simulink model "spike_generator"  (R2020b)
settings: Solver=FixedStepDiscrete  StartTime=0.0  StopTime=stopTime  RelTol=1e-3
InitFcn:
  | initCallback
StopFcn:
  | stopCallback
values from neighbouring files (symbols this model uses):
  nSites = 4    [modelparameters.m]
  t_rd_init = t_rd_rest + 0.02e-3*spont - t_rd_jump    (= 0.0156)    [modelparameters.m]
  t_rd_jump = 0.4e-3    (= 0.0004)    [modelparameters.m]
  t_rd_rest = 14.0e-3    (= 0.014)    [modelparameters.m]
  tabs = 10e-3    (= 0.01)    [modelparameters.m]
  tau = 60e-3    (= 0.06)    [modelparameters.m]
  tdres = 1/Fs    (= 2.08333333333e-05)    [modelparameters.m]
  trel = 10e-3    (= 0.01)    [modelparameters.m]
undefined symbols (not defined in the file or in its folder): mp
libraries: hdlsllib x13
settings Model: Creator=Ross  LastModifiedBy=tyler
settings SolverCC: AutoInsertRateTranBlk=on
settings DataIOCC: SaveOutput=off  SaveTime=off  ReturnWorkspaceOutputs=off
settings OptimizationCC: BlockReduction=off  ConditionallyExecuteInputs=off  DefaultParameterBehavior=Inlined
settings DebuggingCC: ReadBeforeWriteMsg=DisableAll  WriteAfterWriteMsg=DisableAll  WriteAfterReadMsg=DisableAll  AlgebraicLoopMsg=error  MultiTaskDSMMsg=none  SingleTaskRateTransMsg=error  PregeneratedLibrarySubsystemCodeDiagnostic=none  ArithmeticOperatorsInVariantConditions=warning
settings HardwareCC: ProdBitPerPointer=32  ProdBitPerSizeT=32  ProdBitPerPtrDiffT=32  ProdLargestAtomicFloat=None  ProdIntDivRoundTo=Undefined  ProdEndianess=Unspecified  ProdWordSize=32  ProdHWDeviceType=ASIC/FPGA->ASIC/FPGA  TargetBitPerPointer=64  TargetBitPerSizeT=64  TargetBitPerPtrDiffT=64  TargetLongLongMode=on  TargetIntDivRoundTo=Zero  TargetEndianess=LittleEndian  TargetWordSize=64  TargetHWDeviceType=Custom Processor->MATLAB Host Computer  ProdEqTarget=off
settings ModelReferenceCC: UpdateModelReferenceTargets=IfOutOfDate  ModelReferenceNumInstancesAllowed=Single
settings SFSimCC: SFSimEcho=off  SimUseLocalCustomCode=off  CustomCodeUndefinedFunction=UseInterfaceOnly
settings RTWCC: RTWUseLocalCustomCode=off

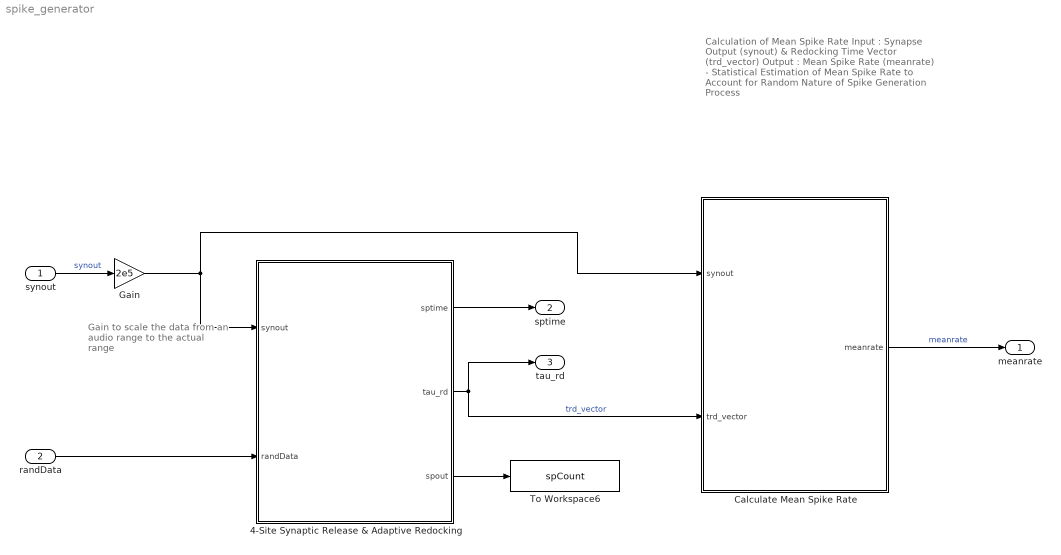
== system spike_generator ==
  note: Gain to scale the
      | data from an audio
      | range to the actual
      | range
  note: Calculation of Mean Spike Rate
      |
      | Input : Synapse Output (synout) & Redocking Time Vector (trd_vector)
      |
      | Output : Mean Spike Rate (meanrate)
      |
      | - Statistical Estimation of Mean Spike Rate to Account for Random Nature of Spike Generation Process
  synout : Inport  OutDataTypeStr=single  PortDimensions=1  SampleTime=[2.0833333333333333e-05,0]
  randData : Inport  Port=2  OutDataTypeStr=single  PortDimensions=[1 1]  SampleTime=[2.0833333333333333e-05,0]
  4-Site Synaptic Release & Adaptive Redocking : Subsystem
  Calculate Mean Spike Rate : Subsystem
  Gain : Gain  Gain=2e5
  To Workspace6 : ToWorkspace  VariableName=spCount  SampleTime=-1
      settings: Save2DSignal=2-D array (concatenate along first dimension)
  meanrate : Outport  OutDataTypeStr=single  PortDimensions=1  SampleTime=[2.0833333333333333e-05,0]
  sptime : Outport  Port=2  OutDataTypeStr=single  PortDimensions=1  SampleTime=[2.0833333333333333e-05,0]
  tau_rd : Outport  Port=3  OutDataTypeStr=single  PortDimensions=1  SampleTime=[2.0833333333333333e-05,0]
  wires:
  4-Site Synaptic Release & Adaptive Redocking/2(tau_rd) -> Calculate Mean Spike Rate/2(trd_vector), tau_rd/1  "trd_vector"
  Calculate Mean Spike Rate/1(meanrate) -> meanrate/1  "meanrate"
  randData/1 -> 4-Site Synaptic Release & Adaptive Redocking/2(randData)
  4-Site Synaptic Release & Adaptive Redocking/1(sptime) -> sptime/1
  synout/1 -> Gain/1  "synout"
  Gain/1 -> 4-Site Synaptic Release & Adaptive Redocking/1(synout), Calculate Mean Spike Rate/1(synout)
  4-Site Synaptic Release & Adaptive Redocking/3(spout) -> To Workspace6/1

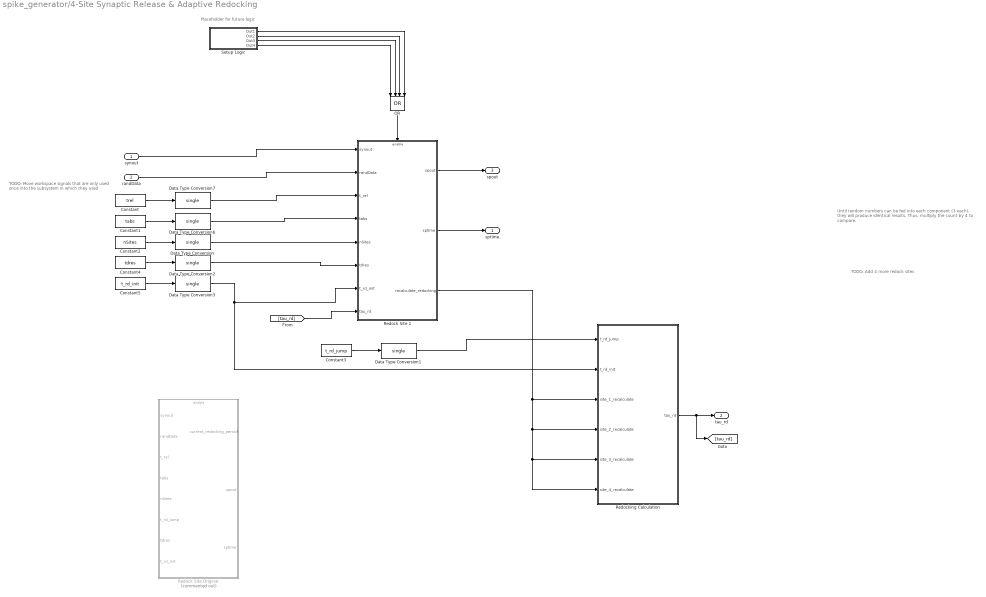
== system spike_generator/4-Site Synaptic Release & Adaptive Redocking ==
  note: TODO: Add 4 more redock sites
  note: Until random numbers can be fed into each component (3 each),
      |  they will produce identical results.  Thus, multiply the count by
      | 4 to compare.
  note: TODO: Move workspace signals that are only
      | used once into the subsystem in which they
      | used
  note: Placeholder for future logic
  synout : Inport
  randData : Inport  Port=2
  Constant : Constant  Value=trel  SampleTime=mp.Ts_sim
  Constant1 : Constant  Value=tabs  SampleTime=mp.Ts_sim
  Constant2 : Constant  Value=nSites  SampleTime=mp.Ts_sim
  Constant3 : Constant  Value=t_rd_jump  SampleTime=mp.Ts_sim
  Constant4 : Constant  Value=tdres  SampleTime=mp.Ts_sim
  Constant5 : Constant  Value=t_rd_init  SampleTime=mp.Ts_sim
  Data Type Conversion{,1..3,6..7} (6 alike) : DataTypeConversion  OutDataTypeStr=single  RndMeth=Nearest
  OR : Logic  Operator=OR  Inputs=4  IconShape=distinctive  AllPortsSameDT=off  OutDataTypeStr=boolean
  Redock Site 1 : Subsystem  TreatAsAtomicUnit=on
  Redock Site Original : Subsystem  Commented=on  TreatAsAtomicUnit=on
  Redocking Calculation : Subsystem
  Setup Logic : Subsystem
  sptime : Outport
  tau_rd : Outport  Port=2
  spout : Outport  Port=3
  wires:
  Setup Logic/1(Out1) -> OR/4
  Setup Logic/2(Out2) -> OR/3
  Setup Logic/3(Out3) -> OR/2
  Setup Logic/4(Out4) -> OR/1
  OR/1 -> Redock Site 1/Enable
  Constant5/1 -> Data Type Conversion3/1
  Constant4/1 -> Data Type Conversion2/1
  Constant3/1 -> Data Type Conversion1/1
  Constant2/1 -> Data Type Conversion/1
  Constant1/1 -> Data Type Conversion6/1
  Data Type Conversion6/1 -> Redock Site 1/4(tabs)
  Data Type Conversion7/1 -> Redock Site 1/3(t_rel)
  Constant/1 -> Data Type Conversion7/1
  Data Type Conversion3/1 -> Redocking Calculation/2(t_rd_init), Redock Site 1/7(t_rd_init)
  Data Type Conversion2/1 -> Redock Site 1/6(tdres)
  Data Type Conversion1/1 -> Redocking Calculation/1(t_rd_jump)
  Data Type Conversion/1 -> Redock Site 1/5(nSites)
  randData/1 -> Redock Site 1/2(randData)
  synout/1 -> Redock Site 1/1(synout)
  Redock Site 1/2(sptime) -> sptime/1
  Redock Site 1/1(spout) -> spout/1
  Redocking Calculation/1(tau_rd) -> tau_rd/1, [tau_rd]
  [tau_rd] -> Redock Site 1/8(tau_rd)
  Redock Site 1/3(recalculate_redocking) -> Redocking Calculation/5(site_3_recalculate), Redocking Calculation/6(site_4_recalculate), Redocking Calculation/4(site_2_recalculate), Redocking Calculation/3(site_1_recalculate)

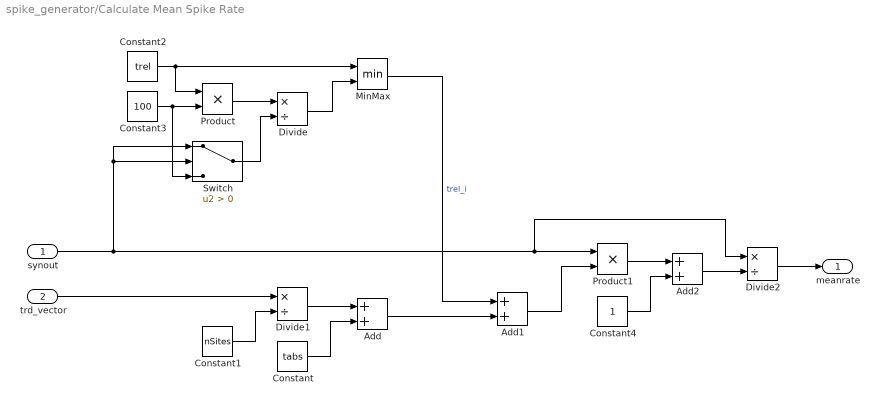
== system spike_generator/Calculate Mean Spike Rate ==
  synout : Inport
  trd_vector : Inport  Port=2
  Add : Sum
  Add1 : Sum
  Add2 : Sum
  Constant : Constant  Value=tabs  OutDataTypeStr=single  SampleTime=-1
  Constant1 : Constant  Value=nSites  OutDataTypeStr=single  SampleTime=-1
  Constant2 : Constant  Value=trel  OutDataTypeStr=single  SampleTime=-1
  Constant3 : Constant  Value=100  OutDataTypeStr=single  SampleTime=-1
  Constant4 : Constant  OutDataTypeStr=single  SampleTime=-1
  Divide : Product  Inputs=*/  RndMeth=Zero  SaturateOnIntegerOverflow=on
  Divide1 : Product  Inputs=*/  RndMeth=Zero  SaturateOnIntegerOverflow=on
  Divide2 : Product  Inputs=*/  RndMeth=Zero  SaturateOnIntegerOverflow=on
  MinMax : MinMax  Inputs=2
  Product : Product
  Product1 : Product
  Switch : Switch  Criteria=u2 > Threshold
  meanrate : Outport  VectorParamsAs1DForOutWhenUnconnected=off
  wires:
  Switch/1 -> Divide/2
  Divide2/1 -> meanrate/1
  Add2/1 -> Divide2/2
  Product1/1 -> Add2/1
  Add1/1 -> Product1/2
  Constant4/1 -> Add2/2
  Add/1 -> Add1/2
  Constant/1 -> Add/2
  Divide1/1 -> Add/1
  Constant1/1 -> Divide1/2
  MinMax/1 -> Add1/1  "trel_i"
  Divide/1 -> MinMax/2
  Product/1 -> Divide/1
  Constant3/1 -> Product/2, Switch/3
  Constant2/1 -> Product/1, MinMax/1
  trd_vector/1 -> Divide1/1
  synout/1 -> Product1/1, Divide2/1, Switch/2, Switch/1

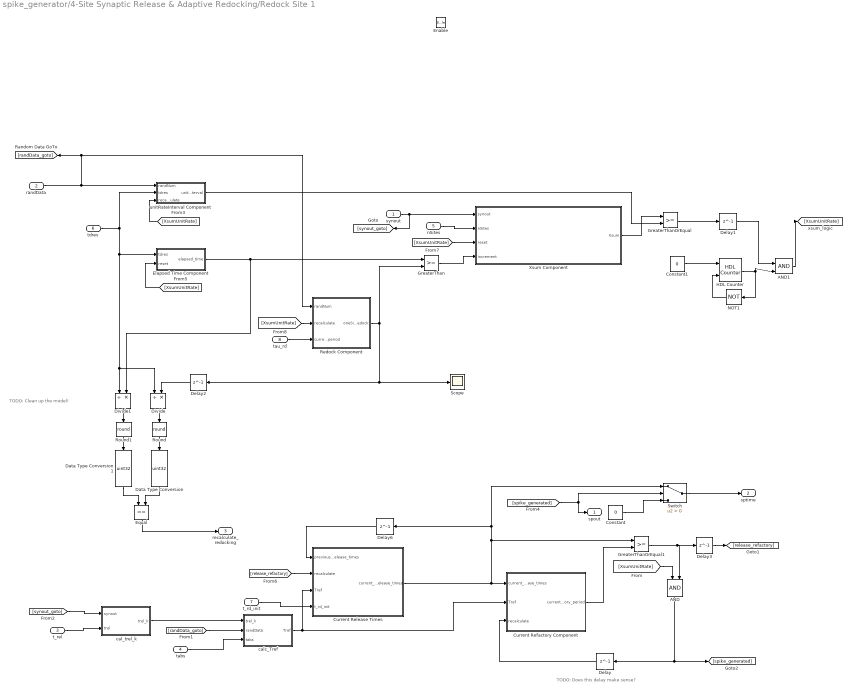
== system spike_generator/4-Site Synaptic Release & Adaptive Redocking/Redock Site 1 ==
  note: TODO: Clean up the model!
  note: TODO: Does this delay make sense?
  synout : Inport
  randData : Inport  Port=2
  t_rel : Inport  Port=3
  tabs : Inport  Port=4
  nSites : Inport  Port=5
  tdres : Inport  Port=6
  t_rd_init : Inport  Port=7
  tau_rd : Inport  Port=8
  Enable : EnablePort
  AND : Logic  IconShape=distinctive  AllPortsSameDT=off  OutDataTypeStr=boolean
  AND1 : Logic  IconShape=distinctive  AllPortsSameDT=off  OutDataTypeStr=boolean
  Constant : Constant  Value=0  OutDataTypeStr=single  SampleTime=-1
  Constant1 : Constant  Value=0  OutDataTypeStr=boolean  SampleTime=-1
  Current Refactory Component : Subsystem
  Current Release Times : Subsystem
  Data Type Conversion : DataTypeConversion  OutDataTypeStr=uint32
  Data Type Conversion1 : DataTypeConversion  OutDataTypeStr=uint32
  Delay{,1..3,6} (5 alike) : Delay  DelayLength=1
  Divide : Product  Inputs=/*
  Divide1 : Product  Inputs=/*
  Elapsed Time Component : Subsystem
  Equal : RelationalOperator  Operator===  OutDataTypeStr=boolean  RndMeth=Simplest
  GreaterThan : RelationalOperator  OutDataTypeStr=boolean  RndMeth=Simplest
  GreaterThanOrEqual : RelationalOperator  OutDataTypeStr=boolean  RndMeth=Simplest
  GreaterThanOrEqual1 : RelationalOperator  OutDataTypeStr=boolean  RndMeth=Simplest
  HDL Counter : hdlsllib/Sources/HDL Counter  CountType=Count limited  CountInit=0  CountStep=1  CountMax=1  CountFromType=Initial value  CountFrom=0  CountResetPort=on  CountLoadPort=off  CountEnbPort=on  CountDirPort=off  CountDataType=Unsigned  CountWordLen=1  CountFracLen=0  CountSampTime=-1
  NOT1 : Logic  Operator=NOT  IconShape=distinctive  AllPortsSameDT=off  OutDataTypeStr=boolean
  Redock Component : Subsystem
  Round : Rounding  Operator=round
  Round1 : Rounding  Operator=round
  Scope : Scope
  Switch : Switch  Criteria=u2 > Threshold
  Xsum Component : Subsystem
  cal_trel_k : Subsystem
  calc_Tref : Subsystem
  unitRateInterval Component : Subsystem
  spout : Outport  InitialOutput=0
  sptime : Outport  Port=2  InitialOutput=0
  recalculate_redocking : Outport  Port=3
  wires:
  Delay2/1 -> Divide/2
  Delay/1 -> Current Refactory Component/3(recalculate)
  GreaterThanOrEqual/1 -> Delay1/1
  AND/1 -> [spike_generated], Delay/1
  [XsumUnitRate] -> Redock Component/2(recalculate)
  GreaterThan/1 -> Xsum Component/4(increment)
  GreaterThanOrEqual1/1 -> Delay3/1, AND/2
  [XsumUnitRate] -> Xsum Component/3(reset)
  [release_refactory] -> Current Release Times/2(recalculate)
  Constant/1 -> Switch/3
  [spike_generated] -> Switch/2, spout/1
  Switch/1 -> sptime/1
  [XsumUnitRate] -> unitRateInterval Component/3(recalculate)
  [synout_goto] -> cal_trel_k/1(synout)
  [randData_goto] -> calc_Tref/2(randData)
  [XsumUnitRate] -> AND/1
  t_rel/1 -> cal_trel_k/2(trel)
  calc_Tref/1(Tref) -> Current Release Times/3(Tref), Current Refactory Component/2(Tref)
  tabs/1 -> calc_Tref/3(tabs)
  cal_trel_k/1(trel_k) -> calc_Tref/1(trel_k)
  Current Refactory Component/1(current_refactory_period) -> GreaterThanOrEqual1/2
  Round1/1 -> Data Type Conversion1/1
  Data Type Conversion1/1 -> Equal/1
  Data Type Conversion/1 -> Equal/2
  Round/1 -> Data Type Conversion/1
  Divide/1 -> Round/1
  Divide1/1 -> Round1/1
  Redock Component/1(oneSiteRedock) -> GreaterThan/2, Scope/1, Delay2/1
  Elapsed Time Component/1(elapsed_time) -> GreaterThan/1, Divide1/2
  Current Release Times/1(current_release_times) -> Current Refactory Component/1(current_release_times), Switch/1, Delay6/1, GreaterThanOrEqual1/1
  nSites/1 -> Xsum Component/2(nSites)
  t_rd_init/1 -> Current Release Times/4(t_rd_init)
  synout/1 -> Xsum Component/1(synout), [synout_goto]
  randData/1 -> Redock Component/1(randNum), [randData_goto], unitRateInterval Component/1(randNum)
  tdres/1 -> Divide/1, Divide1/1, Elapsed Time Component/1(tdres), unitRateInterval Component/2(tdres)
  [XsumUnitRate] -> Elapsed Time Component/2(reset)
  Xsum Component/1(Xsum) -> GreaterThanOrEqual/1
  Delay6/1 -> Current Release Times/1(previous_release_times)
  Delay3/1 -> [release_refactory]
  tau_rd/1 -> Redock Component/3(current_redocking_period)
  Equal/1 -> recalculate_redocking/1
  unitRateInterval Component/1(unitRateInterval) -> GreaterThanOrEqual/2
  NOT1/1 -> HDL Counter/2
  HDL Counter/1 -> AND1/2, NOT1/1
  Constant1/1 -> HDL Counter/1
  Delay1/1 -> AND1/1
  AND1/1 -> [XsumUnitRate]

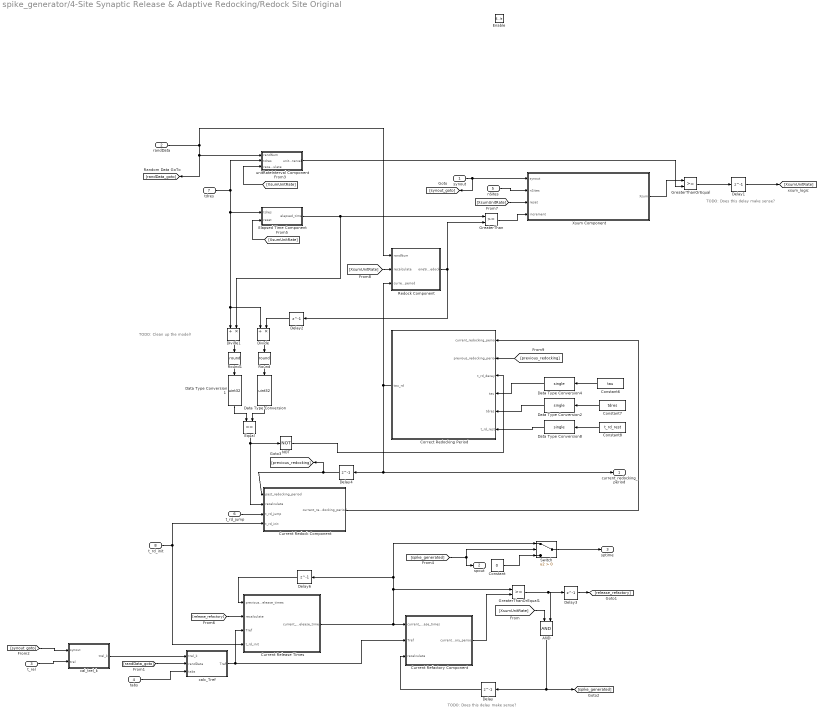
== system spike_generator/4-Site Synaptic Release & Adaptive Redocking/Redock Site Original ==
  note: TODO: Clean up the model!
  note: TODO: Does this delay make sense?
  note: TODO: Does this delay make sense?
  synout : Inport
  randData : Inport  Port=2
  t_rel : Inport  Port=3
  tabs : Inport  Port=4
  nSites : Inport  Port=5
  t_rd_jump : Inport  Port=6
  tdres : Inport  Port=7
  t_rd_init : Inport  Port=8
  Enable : EnablePort
  AND : Logic  IconShape=distinctive  AllPortsSameDT=off  OutDataTypeStr=boolean
  Constant : Constant  Value=0  OutDataTypeStr=single  SampleTime=-1
  Constant6 : Constant  Value=tau  SampleTime=mp.Ts_sim
  Constant7 : Constant  Value=tdres  SampleTime=mp.Ts_sim
  Constant8 : Constant  Value=t_rd_rest  SampleTime=-1
  Correct Redocking Period : Subsystem
  Current Redock Component : Subsystem
  Current Refactory Component : Subsystem
  Current Release Times : Subsystem
  Data Type Conversion : DataTypeConversion  OutDataTypeStr=uint32
  Data Type Conversion1 : DataTypeConversion  OutDataTypeStr=uint32
  Data Type Conversion2 : DataTypeConversion  OutDataTypeStr=single  RndMeth=Nearest
  Data Type Conversion4 : DataTypeConversion  OutDataTypeStr=single  RndMeth=Nearest
  Data Type Conversion8 : DataTypeConversion  OutDataTypeStr=single  RndMeth=Nearest
  Delay{,1..4,6} (6 alike) : Delay  DelayLength=1
  Divide : Product  Inputs=/*
  Divide1 : Product  Inputs=/*
  Elapsed Time Component : Subsystem
  Equal : RelationalOperator  Operator===  OutDataTypeStr=boolean  RndMeth=Simplest
  GreaterThan : RelationalOperator  OutDataTypeStr=boolean  RndMeth=Simplest
  GreaterThanOrEqual : RelationalOperator  OutDataTypeStr=boolean  RndMeth=Simplest
  GreaterThanOrEqual1 : RelationalOperator  OutDataTypeStr=boolean  RndMeth=Simplest
  NOT : Logic  Operator=NOT  IconShape=distinctive  AllPortsSameDT=off  OutDataTypeStr=boolean
  Redock Component : Subsystem
  Round : Rounding  Operator=round
  Round1 : Rounding  Operator=round
  Switch : Switch  Criteria=u2 > Threshold
  Xsum Component : Subsystem
  cal_trel_k : Subsystem
  calc_Tref : Subsystem
  unitRateInterval Component : Subsystem
  current_redocking_period : Outport  InitialOutput=0
  spout : Outport  Port=2  InitialOutput=0
  sptime : Outport  Port=3  InitialOutput=0
  wires:
  Delay2/1 -> Divide/2
  Delay1/1 -> [XsumUnitRate]
  Delay/1 -> Current Refactory Component/3(recalculate)
  GreaterThanOrEqual/1 -> Delay1/1
  AND/1 -> [spike_generated], Delay/1
  [XsumUnitRate] -> Redock Component/2(recalculate)
  GreaterThan/1 -> Xsum Component/4(increment)
  GreaterThanOrEqual1/1 -> Delay3/1, AND/2
  [XsumUnitRate] -> Xsum Component/3(reset)
  [release_refactory] -> Current Release Times/2(recalculate)
  Constant/1 -> Switch/3
  [spike_generated] -> Switch/2, spout/1
  Switch/1 -> sptime/1
  [XsumUnitRate] -> unitRateInterval Component/3(recalculate)
  [synout_goto] -> cal_trel_k/1(synout)
  [randData_goto] -> calc_Tref/2(randData)
  [XsumUnitRate] -> AND/1
  t_rel/1 -> cal_trel_k/2(trel)
  calc_Tref/1(Tref) -> Current Release Times/3(Tref), Current Refactory Component/2(Tref)
  tabs/1 -> calc_Tref/3(tabs)
  cal_trel_k/1(trel_k) -> calc_Tref/1(trel_k)
  Current Refactory Component/1(current_refactory_period) -> GreaterThanOrEqual1/2
  Round1/1 -> Data Type Conversion1/1
  Data Type Conversion1/1 -> Equal/1
  Data Type Conversion/1 -> Equal/2
  Round/1 -> Data Type Conversion/1
  Divide/1 -> Round/1
  Divide1/1 -> Round1/1
  unitRateInterval Component/1(unitRateInterval) -> GreaterThanOrEqual/2
  Equal/1 -> NOT/1, Current Redock Component/2(recalculate)
  Redock Component/1(oneSiteRedock) -> GreaterThan/2, Delay2/1
  Elapsed Time Component/1(elapsed_time) -> GreaterThan/1, Divide1/2
  Current Release Times/1(current_release_times) -> Current Refactory Component/1(current_release_times), Switch/1, Delay6/1, GreaterThanOrEqual1/1
  nSites/1 -> Xsum Component/2(nSites)
  t_rd_jump/1 -> Current Redock Component/3(t_rd_jump)
  t_rd_init/1 -> Current Redock Component/4(t_rd_init), Current Release Times/4(t_rd_init)
  synout/1 -> Xsum Component/1(synout), [synout_goto]
  randData/1 -> Redock Component/1(randNum), [randData_goto], unitRateInterval Component/1(randNum)
  tdres/1 -> Divide/1, Divide1/1, Elapsed Time Component/1(tdres), unitRateInterval Component/2(tdres)
  Delay4/1 -> Current Redock Component/1(past_redocking_period), [previous_redocking]
  NOT/1 -> Correct Redocking Period/3(t_rd_decay)
  Data Type Conversion8/1 -> Correct Redocking Period/6(t_rd_rest)
  Data Type Conversion2/1 -> Correct Redocking Period/5(tdres)
  Constant6/1 -> Data Type Conversion4/1
  Current Redock Component/1(current_redocking_period) -> Correct Redocking Period/1(current_redocking_period)
  Constant7/1 -> Data Type Conversion2/1
  Data Type Conversion4/1 -> Correct Redocking Period/4(tau)
  Constant8/1 -> Data Type Conversion8/1
  Correct Redocking Period/1(tau_rd) -> Redock Component/3(current_redocking_period), current_redocking_period/1, Delay4/1
  [previous_redocking] -> Correct Redocking Period/2(previous_redocking_period)
  [XsumUnitRate] -> Elapsed Time Component/2(reset)
  Xsum Component/1(Xsum) -> GreaterThanOrEqual/1
  Delay6/1 -> Current Release Times/1(previous_release_times)
  Delay3/1 -> [release_refactory]

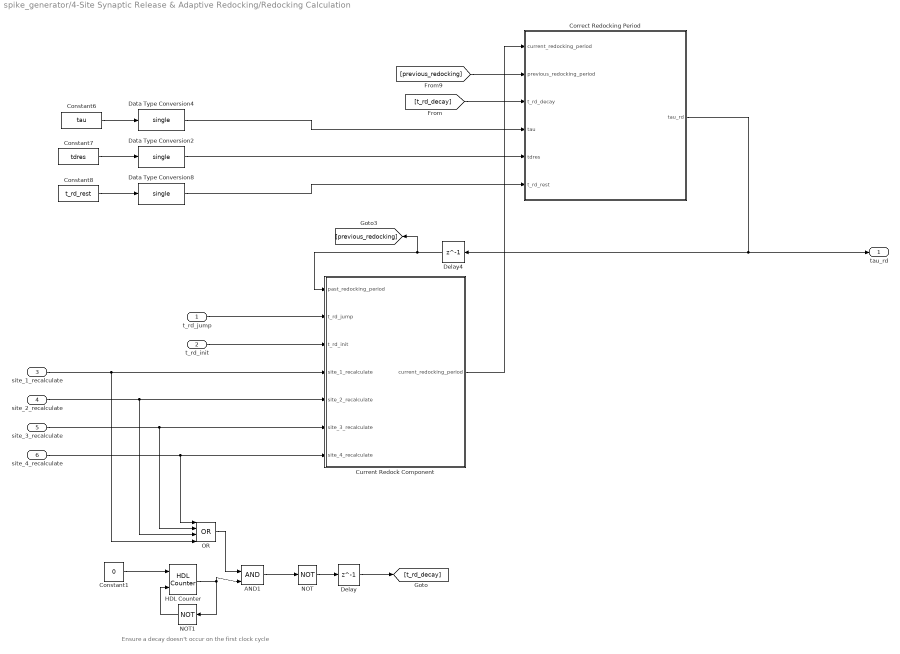
== system spike_generator/4-Site Synaptic Release & Adaptive Redocking/Redocking Calculation ==
  note: Ensure a decay doesn't occur on the first clock cycle
  t_rd_jump : Inport
  t_rd_init : Inport  Port=2
  site_1_recalculate : Inport  Port=3
  site_2_recalculate : Inport  Port=4
  site_3_recalculate : Inport  Port=5
  site_4_recalculate : Inport  Port=6
  AND1 : Logic  IconShape=distinctive  AllPortsSameDT=off  OutDataTypeStr=boolean
  Constant1 : Constant  Value=0  OutDataTypeStr=boolean  SampleTime=-1
  Constant6 : Constant  Value=tau  SampleTime=mp.Ts_sim
  Constant7 : Constant  Value=tdres  SampleTime=mp.Ts_sim
  Constant8 : Constant  Value=t_rd_rest  SampleTime=-1
  Correct Redocking Period : Subsystem
  Current Redock Component : Subsystem
  Data Type Conversion2 : DataTypeConversion  OutDataTypeStr=single  RndMeth=Nearest
  Data Type Conversion4 : DataTypeConversion  OutDataTypeStr=single  RndMeth=Nearest
  Data Type Conversion8 : DataTypeConversion  OutDataTypeStr=single  RndMeth=Nearest
  Delay : Delay  DelayLength=1
  Delay4 : Delay  DelayLength=1
  HDL Counter : hdlsllib/Sources/HDL Counter  CountType=Count limited  CountInit=0  CountStep=1  CountMax=1  CountFromType=Initial value  CountFrom=0  CountResetPort=on  CountLoadPort=off  CountEnbPort=on  CountDirPort=off  CountDataType=Unsigned  CountWordLen=1  CountFracLen=0  CountSampTime=-1
  NOT : Logic  Operator=NOT  IconShape=distinctive  AllPortsSameDT=off  OutDataTypeStr=boolean
  NOT1 : Logic  Operator=NOT  IconShape=distinctive  AllPortsSameDT=off  OutDataTypeStr=boolean
  OR : Logic  Operator=OR  Inputs=4  IconShape=distinctive  AllPortsSameDT=off  OutDataTypeStr=boolean
  tau_rd : Outport  InitialOutput=0
  wires:
  t_rd_init/1 -> Current Redock Component/3(t_rd_init)
  Delay4/1 -> Current Redock Component/1(past_redocking_period), [previous_redocking]
  Constant8/1 -> Data Type Conversion8/1
  t_rd_jump/1 -> Current Redock Component/2(t_rd_jump)
  Current Redock Component/1(current_redocking_period) -> Correct Redocking Period/1(current_redocking_period)
  Data Type Conversion4/1 -> Correct Redocking Period/4(tau)
  Data Type Conversion8/1 -> Correct Redocking Period/6(t_rd_rest)
  Correct Redocking Period/1(tau_rd) -> Delay4/1, tau_rd/1
  site_1_recalculate/1 -> OR/4, Current Redock Component/4(site_1_recalculate)
  Constant7/1 -> Data Type Conversion2/1
  Data Type Conversion2/1 -> Correct Redocking Period/5(tdres)
  Constant6/1 -> Data Type Conversion4/1
  [previous_redocking] -> Correct Redocking Period/2(previous_redocking_period)
  site_2_recalculate/1 -> OR/3, Current Redock Component/5(site_2_recalculate)
  site_3_recalculate/1 -> OR/2, Current Redock Component/6(site_3_recalculate)
  site_4_recalculate/1 -> OR/1, Current Redock Component/7(site_4_recalculate)
  [t_rd_decay] -> Correct Redocking Period/3(t_rd_decay)
  NOT/1 -> Delay/1
  Delay/1 -> [t_rd_decay]
  Constant1/1 -> HDL Counter/1
  OR/1 -> AND1/1
  HDL Counter/1 -> AND1/2, NOT1/1
  AND1/1 -> NOT/1
  NOT1/1 -> HDL Counter/2

== system spike_generator/4-Site Synaptic Release & Adaptive Redocking/Setup Logic ==
  Constant : Constant  OutDataTypeStr=boolean  SampleTime=-1
  Out1 : Outport
  Out2 : Outport  Port=2
  Out3 : Outport  Port=3
  Out4 : Outport  Port=4
  wires:
  Constant/1 -> Out4/1, Out3/1, Out2/1, Out1/1

== system spike_generator/4-Site Synaptic Release & Adaptive Redocking/Redock Site 1/Current Refactory Component ==
  current_release_times : Inport
  Tref : Inport  Port=2
  recalculate : Inport  Port=3
  Add : Sum
  Constant : Constant  Value=0  OutDataTypeStr=single  SampleTime=-1
  Delay : Delay  DelayLength=1
  Initialization Signal : Subsystem
  Switch : Switch  Criteria=u2 > Threshold  OutDataTypeStr=single
  Switch1 : Switch  Criteria=u2 ~= 0  OutDataTypeStr=single
  current_refactory_period : Outport
  wires:
  Delay/1 -> Switch1/3
  Switch/1 -> current_refactory_period/1, Delay/1
  Switch1/1 -> Switch/3
  Add/1 -> Switch1/1
  current_release_times/1 -> Add/1
  Tref/1 -> Add/2
  recalculate/1 -> Switch1/2
  Initialization Signal/1(initalize) -> Switch/2
  Constant/1 -> Switch/1

== system spike_generator/4-Site Synaptic Release & Adaptive Redocking/Redock Site 1/Current Release Times ==
  previous_release_times : Inport
  recalculate : Inport  Port=2
  Tref : Inport  Port=3
  t_rd_init : Inport  Port=4
  Add : Sum
  Delay : Delay  DelayLength=1
  Initialization Signal : Subsystem
  Switch : Switch  Criteria=u2 > Threshold  OutDataTypeStr=single
  Switch1 : Switch  Criteria=u2 ~= 0  OutDataTypeStr=single
  current_release_times : Outport
  wires:
  Delay/1 -> Switch1/3
  Switch/1 -> current_release_times/1, Delay/1
  Switch1/1 -> Switch/3
  recalculate/1 -> Switch1/2
  Add/1 -> Switch1/1
  previous_release_times/1 -> Add/1
  Tref/1 -> Add/2
  Initialization Signal/1(initalize) -> Switch/2
  t_rd_init/1 -> Switch/1

== system spike_generator/4-Site Synaptic Release & Adaptive Redocking/Redock Site 1/Elapsed Time Component ==
  tdres : Inport
  reset : Inport  Port=2
  Data Type Conversion : DataTypeConversion  OutDataTypeStr=boolean
  Data Type Conversion1 : DataTypeConversion  OutDataTypeStr=single
  HDL Counter : hdlsllib/Sources/HDL Counter  CountType=Count limited  CountInit=0  CountStep=1  CountMax=1023  CountFromType=Initial value  CountFrom=0  CountResetPort=on  CountLoadPort=off  CountEnbPort=off  CountDirPort=off  CountDataType=Unsigned  CountWordLen=10  CountFracLen=0  CountSampTime=-1
  Product : Product  OutDataTypeStr=single
  elapsed_time : Outport
  wires:
  Data Type Conversion1/1 -> Product/2
  Data Type Conversion/1 -> HDL Counter/1
  Product/1 -> elapsed_time/1
  tdres/1 -> Product/1
  HDL Counter/1 -> Data Type Conversion1/1
  reset/1 -> Data Type Conversion/1

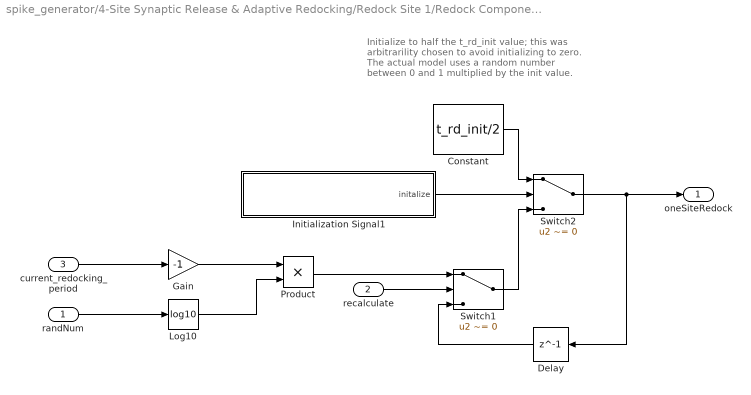
== system spike_generator/4-Site Synaptic Release & Adaptive Redocking/Redock Site 1/Redock Component ==
  note: Initialize to half the t_rd_init value; this was
      | arbitrarility chosen to avoid initializing to zero.
      | The actual model uses a random number
      | between 0 and 1 multiplied by the init value.
  randNum : Inport
  recalculate : Inport  Port=2
  current_redocking_period : Inport  Port=3
  Constant : Constant  Value=t_rd_init/2  OutDataTypeStr=single  SampleTime=-1
  Delay : Delay  DelayLength=1
  Gain : Gain  Gain=-1
  Initialization Signal1 : Subsystem
  Log10 : Math  Operator=log10  SaturateOnIntegerOverflow=on
  Product : Product
  Switch1 : Switch  Criteria=u2 ~= 0  OutDataTypeStr=single
  Switch2 : Switch  Criteria=u2 ~= 0  OutDataTypeStr=single
  oneSiteRedock : Outport
  wires:
  Delay/1 -> Switch1/3
  Switch1/1 -> Switch2/3
  Initialization Signal1/1(initalize) -> Switch2/2
  Constant/1 -> Switch2/1
  Switch2/1 -> oneSiteRedock/1, Delay/1
  Log10/1 -> Product/2
  Gain/1 -> Product/1
  current_redocking_period/1 -> Gain/1
  Product/1 -> Switch1/1
  randNum/1 -> Log10/1
  recalculate/1 -> Switch1/2

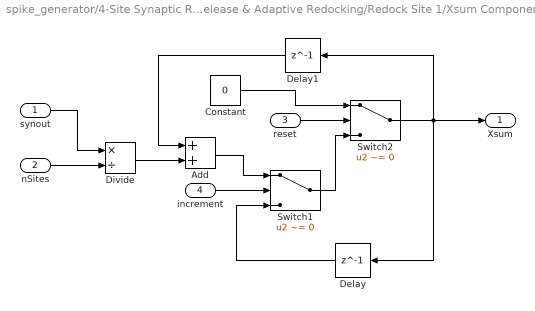
== system spike_generator/4-Site Synaptic Release & Adaptive Redocking/Redock Site 1/Xsum Component ==
  synout : Inport
  nSites : Inport  Port=2
  reset : Inport  Port=3
  increment : Inport  Port=4
  Add : Sum
  Constant : Constant  Value=0  OutDataTypeStr=single  SampleTime=-1
  Delay : Delay  DelayLength=1
  Delay1 : Delay  DelayLength=1
  Divide : Product  Inputs=*/
  Switch1 : Switch  Criteria=u2 ~= 0  OutDataTypeStr=single
  Switch2 : Switch  Criteria=u2 ~= 0  OutDataTypeStr=single
  Xsum : Outport
  wires:
  Delay1/1 -> Add/1
  Delay/1 -> Switch1/3
  Switch2/1 -> Xsum/1, Delay1/1, Delay/1
  Add/1 -> Switch1/1
  Divide/1 -> Add/2
  nSites/1 -> Divide/2
  synout/1 -> Divide/1
  Constant/1 -> Switch2/1
  Switch1/1 -> Switch2/3
  increment/1 -> Switch1/2
  reset/1 -> Switch2/2

== system spike_generator/4-Site Synaptic Release & Adaptive Redocking/Redock Site 1/cal_trel_k ==
  synout : Inport
  trel : Inport  Port=2
  Divide : Product  Inputs=*/
  K : Gain  Gain=100
  Min : MinMax  Inputs=2
  trel_k : Outport
  wires:
  synout/1 -> Divide/2
  trel/1 -> Min/2, K/1
  K/1 -> Divide/1
  Min/1 -> trel_k/1
  Divide/1 -> Min/1

== system spike_generator/4-Site Synaptic Release & Adaptive Redocking/Redock Site 1/calc_Tref ==
  trel_k : Inport
  randData : Inport  Port=2
  tabs : Inport  Port=3
  Log10 : Math  Operator=log10  SaturateOnIntegerOverflow=on
  Product : Product
  Subtract : Sum  Inputs=+-
  Tref : Outport
  wires:
  Subtract/1 -> Tref/1
  Product/1 -> Subtract/2
  Log10/1 -> Product/2
  trel_k/1 -> Product/1
  randData/1 -> Log10/1
  tabs/1 -> Subtract/1

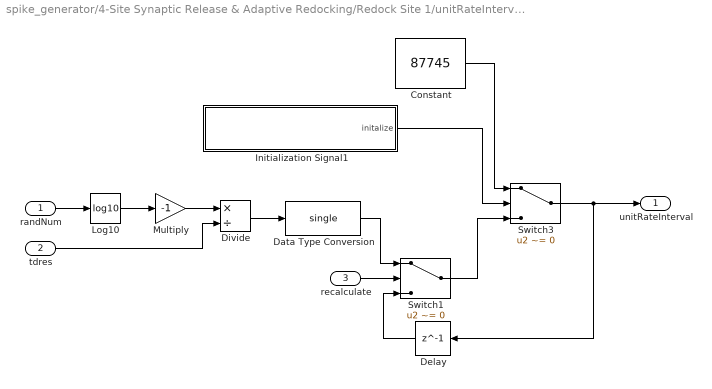
== system spike_generator/4-Site Synaptic Release & Adaptive Redocking/Redock Site 1/unitRateInterval Component ==
  randNum : Inport
  tdres : Inport  Port=2
  recalculate : Inport  Port=3
  Constant : Constant  Value=87745  OutDataTypeStr=single  SampleTime=-1
  Data Type Conversion : DataTypeConversion  OutDataTypeStr=single
  Delay : Delay  DelayLength=1
  Divide : Product  Inputs=*/
  Initialization Signal1 : Subsystem
  Log10 : Math  Operator=log10  SaturateOnIntegerOverflow=on
  Multiply : Gain  Gain=-1
  Switch1 : Switch  Criteria=u2 ~= 0  OutDataTypeStr=single
  Switch3 : Switch  Criteria=u2 ~= 0  OutDataTypeStr=single
  unitRateInterval : Outport
  wires:
  Delay/1 -> Switch1/3
  Switch1/1 -> Switch3/3
  recalculate/1 -> Switch1/2
  randNum/1 -> Log10/1
  Log10/1 -> Multiply/1
  Data Type Conversion/1 -> Switch1/1
  Divide/1 -> Data Type Conversion/1
  tdres/1 -> Divide/2
  Multiply/1 -> Divide/1
  Constant/1 -> Switch3/1
  Switch3/1 -> Delay/1, unitRateInterval/1
  Initialization Signal1/1(initalize) -> Switch3/2

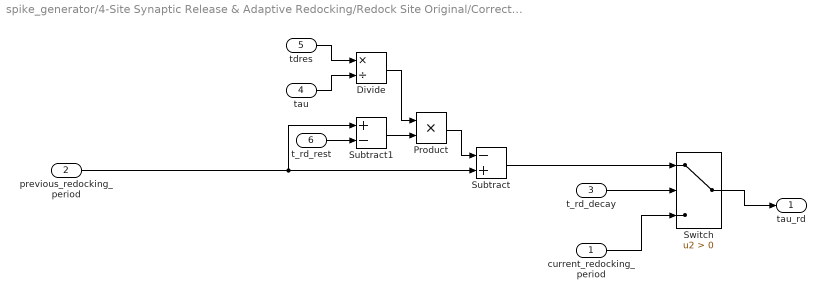
== system spike_generator/4-Site Synaptic Release & Adaptive Redocking/Redock Site Original/Correct Redocking Period ==
  current_redocking_period : Inport
  previous_redocking_period : Inport  Port=2
  t_rd_decay : Inport  Port=3
  tau : Inport  Port=4
  tdres : Inport  Port=5
  t_rd_rest : Inport  Port=6
  Divide : Product  Inputs=*/
  Product : Product
  Subtract : Sum  Inputs=-+
  Subtract1 : Sum  Inputs=+-
  Switch : Switch  Criteria=u2 > Threshold
  tau_rd : Outport
  wires:
  Subtract/1 -> Switch/1
  Product/1 -> Subtract/1
  Subtract1/1 -> Product/2
  Divide/1 -> Product/1
  t_rd_rest/1 -> Subtract1/2
  tau/1 -> Divide/2
  tdres/1 -> Divide/1
  previous_redocking_period/1 -> Subtract/2, Subtract1/1
  Switch/1 -> tau_rd/1
  t_rd_decay/1 -> Switch/2
  current_redocking_period/1 -> Switch/3

== system spike_generator/4-Site Synaptic Release & Adaptive Redocking/Redock Site Original/Current Redock Component ==
  past_redocking_period : Inport
  recalculate : Inport  Port=2
  t_rd_jump : Inport  Port=3
  t_rd_init : Inport  Port=4
  Add : Sum
  Delay : Delay  DelayLength=1
  Initialization Signal : Subsystem
  Switch : Switch  Criteria=u2 ~= 0  OutDataTypeStr=single
  Switch1 : Switch  Criteria=u2 ~= 0  OutDataTypeStr=single
  current_redocking_period : Outport
  wires:
  Delay/1 -> Switch1/3
  Switch/1 -> current_redocking_period/1, Delay/1
  past_redocking_period/1 -> Add/1
  t_rd_jump/1 -> Add/2
  Add/1 -> Switch1/1
  recalculate/1 -> Switch1/2
  Switch1/1 -> Switch/3
  t_rd_init/1 -> Switch/1
  Initialization Signal/1(initalize) -> Switch/2

== system spike_generator/4-Site Synaptic Release & Adaptive Redocking/Redock Site Original/Current Refactory Component ==
  current_release_times : Inport
  Tref : Inport  Port=2
  recalculate : Inport  Port=3
  Add : Sum
  Constant : Constant  Value=0  OutDataTypeStr=single  SampleTime=-1
  Delay : Delay  DelayLength=1
  Initialization Signal : Subsystem
  Switch : Switch  Criteria=u2 > Threshold  OutDataTypeStr=single
  Switch1 : Switch  Criteria=u2 ~= 0  OutDataTypeStr=single
  current_refactory_period : Outport
  wires:
  Delay/1 -> Switch1/3
  Switch/1 -> current_refactory_period/1, Delay/1
  Switch1/1 -> Switch/3
  Add/1 -> Switch1/1
  current_release_times/1 -> Add/1
  Tref/1 -> Add/2
  recalculate/1 -> Switch1/2
  Initialization Signal/1(initalize) -> Switch/2
  Constant/1 -> Switch/1

== system spike_generator/4-Site Synaptic Release & Adaptive Redocking/Redock Site Original/Current Release Times ==
  previous_release_times : Inport
  recalculate : Inport  Port=2
  Tref : Inport  Port=3
  t_rd_init : Inport  Port=4
  Add : Sum
  Delay : Delay  DelayLength=1
  Initialization Signal : Subsystem
  Switch : Switch  Criteria=u2 > Threshold  OutDataTypeStr=single
  Switch1 : Switch  Criteria=u2 ~= 0  OutDataTypeStr=single
  current_release_times : Outport
  wires:
  Delay/1 -> Switch1/3
  Switch/1 -> current_release_times/1, Delay/1
  Switch1/1 -> Switch/3
  recalculate/1 -> Switch1/2
  Add/1 -> Switch1/1
  previous_release_times/1 -> Add/1
  Tref/1 -> Add/2
  Initialization Signal/1(initalize) -> Switch/2
  t_rd_init/1 -> Switch/1

== system spike_generator/4-Site Synaptic Release & Adaptive Redocking/Redock Site Original/Elapsed Time Component ==
  tdres : Inport
  reset : Inport  Port=2
  Data Type Conversion : DataTypeConversion  OutDataTypeStr=boolean
  Data Type Conversion1 : DataTypeConversion  OutDataTypeStr=single
  HDL Counter : hdlsllib/Sources/HDL Counter  CountType=Count limited  CountInit=0  CountStep=1  CountMax=1023  CountFromType=Initial value  CountFrom=0  CountResetPort=on  CountLoadPort=off  CountEnbPort=off  CountDirPort=off  CountDataType=Unsigned  CountWordLen=10  CountFracLen=0  CountSampTime=-1
  Product : Product  OutDataTypeStr=single
  elapsed_time : Outport
  wires:
  Data Type Conversion1/1 -> Product/2
  Data Type Conversion/1 -> HDL Counter/1
  Product/1 -> elapsed_time/1
  tdres/1 -> Product/1
  HDL Counter/1 -> Data Type Conversion1/1
  reset/1 -> Data Type Conversion/1

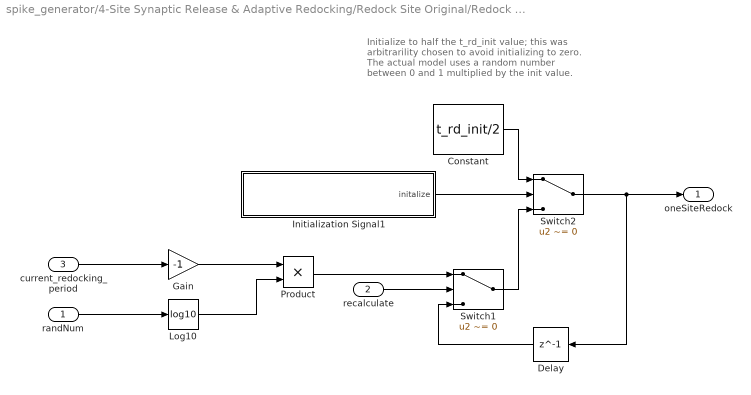
== system spike_generator/4-Site Synaptic Release & Adaptive Redocking/Redock Site Original/Redock Component ==
  note: Initialize to half the t_rd_init value; this was
      | arbitrarility chosen to avoid initializing to zero.
      | The actual model uses a random number
      | between 0 and 1 multiplied by the init value.
  randNum : Inport
  recalculate : Inport  Port=2
  current_redocking_period : Inport  Port=3
  Constant : Constant  Value=t_rd_init/2  OutDataTypeStr=single  SampleTime=-1
  Delay : Delay  DelayLength=1
  Gain : Gain  Gain=-1
  Initialization Signal1 : Subsystem
  Log10 : Math  Operator=log10  SaturateOnIntegerOverflow=on
  Product : Product
  Switch1 : Switch  Criteria=u2 ~= 0  OutDataTypeStr=single
  Switch2 : Switch  Criteria=u2 ~= 0  OutDataTypeStr=single
  oneSiteRedock : Outport
  wires:
  Delay/1 -> Switch1/3
  Switch1/1 -> Switch2/3
  Initialization Signal1/1(initalize) -> Switch2/2
  Constant/1 -> Switch2/1
  Switch2/1 -> oneSiteRedock/1, Delay/1
  Log10/1 -> Product/2
  Gain/1 -> Product/1
  current_redocking_period/1 -> Gain/1
  Product/1 -> Switch1/1
  randNum/1 -> Log10/1
  recalculate/1 -> Switch1/2

== system spike_generator/4-Site Synaptic Release & Adaptive Redocking/Redock Site Original/Xsum Component ==
  synout : Inport
  nSites : Inport  Port=2
  reset : Inport  Port=3
  increment : Inport  Port=4
  Add : Sum
  Constant : Constant  Value=0  OutDataTypeStr=single  SampleTime=-1
  Delay : Delay  DelayLength=1
  Delay1 : Delay  DelayLength=1
  Divide : Product  Inputs=*/
  Switch1 : Switch  Criteria=u2 ~= 0  OutDataTypeStr=single
  Switch2 : Switch  Criteria=u2 ~= 0  OutDataTypeStr=single
  Xsum : Outport
  wires:
  Delay1/1 -> Add/1
  Delay/1 -> Switch1/3
  Switch2/1 -> Xsum/1, Delay1/1, Delay/1
  Add/1 -> Switch1/1
  Divide/1 -> Add/2
  nSites/1 -> Divide/2
  synout/1 -> Divide/1
  Constant/1 -> Switch2/1
  Switch1/1 -> Switch2/3
  increment/1 -> Switch1/2
  reset/1 -> Switch2/2

== system spike_generator/4-Site Synaptic Release & Adaptive Redocking/Redock Site Original/cal_trel_k ==
  synout : Inport
  trel : Inport  Port=2
  Divide : Product  Inputs=*/
  K : Gain  Gain=100
  Min : MinMax  Inputs=2
  trel_k : Outport
  wires:
  synout/1 -> Divide/2
  trel/1 -> Min/2, K/1
  K/1 -> Divide/1
  Min/1 -> trel_k/1
  Divide/1 -> Min/1

== system spike_generator/4-Site Synaptic Release & Adaptive Redocking/Redock Site Original/calc_Tref ==
  trel_k : Inport
  randData : Inport  Port=2
  tabs : Inport  Port=3
  Log10 : Math  Operator=log10  SaturateOnIntegerOverflow=on
  Product : Product
  Subtract : Sum  Inputs=+-
  Tref : Outport
  wires:
  Subtract/1 -> Tref/1
  Product/1 -> Subtract/2
  Log10/1 -> Product/2
  trel_k/1 -> Product/1
  randData/1 -> Log10/1
  tabs/1 -> Subtract/1

== system spike_generator/4-Site Synaptic Release & Adaptive Redocking/Redock Site Original/unitRateInterval Component ==
  randNum : Inport
  tdres : Inport  Port=2
  recalculate : Inport  Port=3
  Data Type Conversion : DataTypeConversion  OutDataTypeStr=single
  Delay : Delay  DelayLength=1
  Divide : Product  Inputs=*/
  Log10 : Math  Operator=log10  SaturateOnIntegerOverflow=on
  Multiply : Gain  Gain=-1
  Switch1 : Switch  Criteria=u2 ~= 0  OutDataTypeStr=single
  unitRateInterval : Outport
  wires:
  Delay/1 -> Switch1/3
  Switch1/1 -> unitRateInterval/1, Delay/1
  recalculate/1 -> Switch1/2
  randNum/1 -> Log10/1
  Log10/1 -> Multiply/1
  Data Type Conversion/1 -> Switch1/1
  Divide/1 -> Data Type Conversion/1
  tdres/1 -> Divide/2
  Multiply/1 -> Divide/1

== system spike_generator/4-Site Synaptic Release & Adaptive Redocking/Redocking Calculation/Correct Redocking Period ==
  current_redocking_period : Inport
  previous_redocking_period : Inport  Port=2
  t_rd_decay : Inport  Port=3
  tau : Inport  Port=4
  tdres : Inport  Port=5
  t_rd_rest : Inport  Port=6
  Divide : Product  Inputs=*/
  Product : Product
  Subtract : Sum  Inputs=-+
  Subtract1 : Sum  Inputs=+-
  Switch : Switch  Criteria=u2 > Threshold
  tau_rd : Outport
  wires:
  Subtract/1 -> Switch/1
  Product/1 -> Subtract/1
  Subtract1/1 -> Product/2
  Divide/1 -> Product/1
  t_rd_rest/1 -> Subtract1/2
  tau/1 -> Divide/2
  tdres/1 -> Divide/1
  previous_redocking_period/1 -> Subtract/2, Subtract1/1
  Switch/1 -> tau_rd/1
  t_rd_decay/1 -> Switch/2
  current_redocking_period/1 -> Switch/3

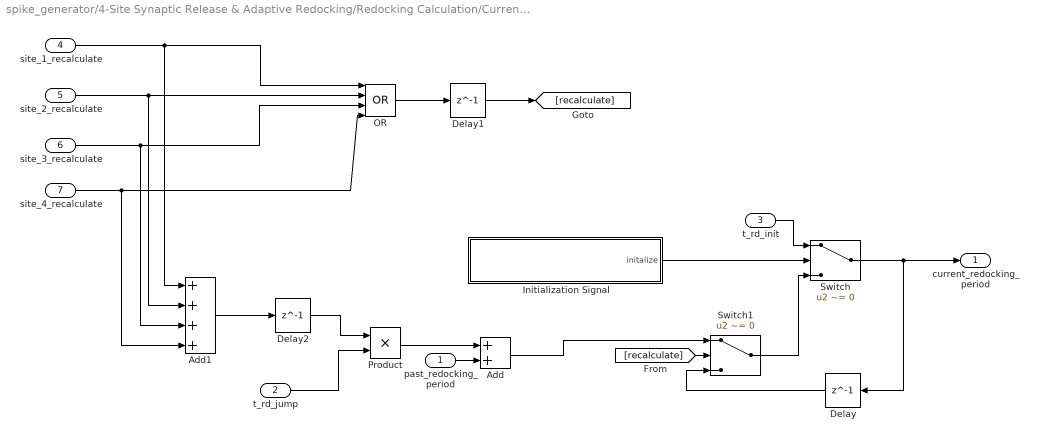
== system spike_generator/4-Site Synaptic Release & Adaptive Redocking/Redocking Calculation/Current Redock Component ==
  past_redocking_period : Inport
  t_rd_jump : Inport  Port=2
  t_rd_init : Inport  Port=3
  site_1_recalculate : Inport  Port=4
  site_2_recalculate : Inport  Port=5
  site_3_recalculate : Inport  Port=6
  site_4_recalculate : Inport  Port=7
  Add : Sum
  Add1 : Sum  Inputs=++++
  Delay : Delay  DelayLength=1
  Delay1 : Delay  DelayLength=1
  Delay2 : Delay  DelayLength=1
  Initialization Signal : Subsystem
  OR : Logic  Operator=OR  Inputs=4  IconShape=distinctive  AllPortsSameDT=off  OutDataTypeStr=boolean
  Product : Product
  Switch : Switch  Criteria=u2 ~= 0  OutDataTypeStr=single
  Switch1 : Switch  Criteria=u2 ~= 0  OutDataTypeStr=single
  current_redocking_period : Outport
  wires:
  Delay/1 -> Switch1/3
  Switch/1 -> current_redocking_period/1, Delay/1
  Add/1 -> Switch1/1
  Switch1/1 -> Switch/3
  t_rd_init/1 -> Switch/1
  Initialization Signal/1(initalize) -> Switch/2
  site_1_recalculate/1 -> Add1/1, OR/1
  site_2_recalculate/1 -> Add1/2, OR/2
  site_3_recalculate/1 -> OR/3, Add1/3
  site_4_recalculate/1 -> OR/4, Add1/4
  [recalculate] -> Switch1/2
  past_redocking_period/1 -> Add/2
  Product/1 -> Add/1
  t_rd_jump/1 -> Product/2
  Add1/1 -> Delay2/1
  OR/1 -> Delay1/1
  Delay1/1 -> [recalculate]
  Delay2/1 -> Product/1

== system spike_generator/4-Site Synaptic Release & Adaptive Redocking/Redock Site 1/Current Refactory Component/Initialization Signal ==
  note: This should probably be a model reference...
  Constant1 : Constant  Value=0  SampleTime=-1
  Constant2 : Constant  SampleTime=-1
  Data Type Conversion : DataTypeConversion  OutDataTypeStr=boolean
  HDL Counter : hdlsllib/Sources/HDL Counter  CountType=Count limited  CountInit=0  CountStep=1  CountMax=2  CountFromType=Initial value  CountFrom=0  CountResetPort=off  CountLoadPort=off  CountEnbPort=on  CountDirPort=off  CountDataType=Unsigned  CountWordLen=2  CountFracLen=0  CountSampTime=-1
  Switch : Switch  Criteria=u2 > Threshold
  initalize : Outport
  wires:
  Data Type Conversion/1 -> HDL Counter/1
  Switch/1 -> initalize/1, Data Type Conversion/1
  HDL Counter/1 -> Switch/2
  Constant2/1 -> Switch/3
  Constant1/1 -> Switch/1

== system spike_generator/4-Site Synaptic Release & Adaptive Redocking/Redock Site 1/Current Release Times/Initialization Signal ==
  note: This should probably be a model reference...
  Constant1 : Constant  Value=0  SampleTime=-1
  Constant2 : Constant  SampleTime=-1
  Data Type Conversion : DataTypeConversion  OutDataTypeStr=boolean
  HDL Counter : hdlsllib/Sources/HDL Counter  CountType=Count limited  CountInit=0  CountStep=1  CountMax=2  CountFromType=Initial value  CountFrom=0  CountResetPort=off  CountLoadPort=off  CountEnbPort=on  CountDirPort=off  CountDataType=Unsigned  CountWordLen=2  CountFracLen=0  CountSampTime=-1
  Switch : Switch  Criteria=u2 > Threshold
  initalize : Outport
  wires:
  Data Type Conversion/1 -> HDL Counter/1
  Switch/1 -> initalize/1, Data Type Conversion/1
  HDL Counter/1 -> Switch/2
  Constant2/1 -> Switch/3
  Constant1/1 -> Switch/1

== system spike_generator/4-Site Synaptic Release & Adaptive Redocking/Redock Site 1/Redock Component/Initialization Signal1 ==
  note: This should probably be a model reference...
  Constant1 : Constant  Value=0  SampleTime=-1
  Constant2 : Constant  SampleTime=-1
  Data Type Conversion : DataTypeConversion  OutDataTypeStr=boolean
  HDL Counter : hdlsllib/Sources/HDL Counter  CountType=Count limited  CountInit=0  CountStep=1  CountMax=2  CountFromType=Initial value  CountFrom=0  CountResetPort=off  CountLoadPort=off  CountEnbPort=on  CountDirPort=off  CountDataType=Unsigned  CountWordLen=2  CountFracLen=0  CountSampTime=-1
  Switch : Switch  Criteria=u2 > Threshold
  initalize : Outport
  wires:
  Data Type Conversion/1 -> HDL Counter/1
  Switch/1 -> initalize/1, Data Type Conversion/1
  HDL Counter/1 -> Switch/2
  Constant2/1 -> Switch/3
  Constant1/1 -> Switch/1

== system spike_generator/4-Site Synaptic Release & Adaptive Redocking/Redock Site 1/unitRateInterval Component/Initialization Signal1 ==
  note: This should probably be a model reference...
  Constant1 : Constant  Value=0  SampleTime=-1
  Constant2 : Constant  SampleTime=-1
  Data Type Conversion : DataTypeConversion  OutDataTypeStr=boolean
  HDL Counter : hdlsllib/Sources/HDL Counter  CountType=Count limited  CountInit=0  CountStep=1  CountMax=2  CountFromType=Initial value  CountFrom=0  CountResetPort=off  CountLoadPort=off  CountEnbPort=on  CountDirPort=off  CountDataType=Unsigned  CountWordLen=2  CountFracLen=0  CountSampTime=-1
  Switch : Switch  Criteria=u2 > Threshold
  initalize : Outport
  wires:
  Data Type Conversion/1 -> HDL Counter/1
  Switch/1 -> initalize/1, Data Type Conversion/1
  HDL Counter/1 -> Switch/2
  Constant2/1 -> Switch/3
  Constant1/1 -> Switch/1

== system spike_generator/4-Site Synaptic Release & Adaptive Redocking/Redock Site Original/Current Redock Component/Initialization Signal ==
  note: This should probably be a model reference...
  Constant1 : Constant  Value=0  SampleTime=-1
  Constant2 : Constant  SampleTime=-1
  Data Type Conversion : DataTypeConversion  OutDataTypeStr=boolean
  HDL Counter : hdlsllib/Sources/HDL Counter  CountType=Count limited  CountInit=0  CountStep=1  CountMax=3  CountFromType=Initial value  CountFrom=0  CountResetPort=off  CountLoadPort=off  CountEnbPort=on  CountDirPort=off  CountDataType=Unsigned  CountWordLen=2  CountFracLen=0  CountSampTime=-1
  Switch : Switch  Criteria=u2 > Threshold
  initalize : Outport
  wires:
  Data Type Conversion/1 -> HDL Counter/1
  Switch/1 -> initalize/1, Data Type Conversion/1
  HDL Counter/1 -> Switch/2
  Constant2/1 -> Switch/3
  Constant1/1 -> Switch/1

== system spike_generator/4-Site Synaptic Release & Adaptive Redocking/Redock Site Original/Current Refactory Component/Initialization Signal ==
  note: This should probably be a model reference...
  Constant1 : Constant  Value=0  SampleTime=-1
  Constant2 : Constant  SampleTime=-1
  Data Type Conversion : DataTypeConversion  OutDataTypeStr=boolean
  HDL Counter : hdlsllib/Sources/HDL Counter  CountType=Count limited  CountInit=0  CountStep=1  CountMax=2  CountFromType=Initial value  CountFrom=0  CountResetPort=off  CountLoadPort=off  CountEnbPort=on  CountDirPort=off  CountDataType=Unsigned  CountWordLen=2  CountFracLen=0  CountSampTime=-1
  Switch : Switch  Criteria=u2 > Threshold
  initalize : Outport
  wires:
  Data Type Conversion/1 -> HDL Counter/1
  Switch/1 -> initalize/1, Data Type Conversion/1
  HDL Counter/1 -> Switch/2
  Constant2/1 -> Switch/3
  Constant1/1 -> Switch/1

== system spike_generator/4-Site Synaptic Release & Adaptive Redocking/Redock Site Original/Current Release Times/Initialization Signal ==
  note: This should probably be a model reference...
  Constant1 : Constant  Value=0  SampleTime=-1
  Constant2 : Constant  SampleTime=-1
  Data Type Conversion : DataTypeConversion  OutDataTypeStr=boolean
  HDL Counter : hdlsllib/Sources/HDL Counter  CountType=Count limited  CountInit=0  CountStep=1  CountMax=2  CountFromType=Initial value  CountFrom=0  CountResetPort=off  CountLoadPort=off  CountEnbPort=on  CountDirPort=off  CountDataType=Unsigned  CountWordLen=2  CountFracLen=0  CountSampTime=-1
  Switch : Switch  Criteria=u2 > Threshold
  initalize : Outport
  wires:
  Data Type Conversion/1 -> HDL Counter/1
  Switch/1 -> initalize/1, Data Type Conversion/1
  HDL Counter/1 -> Switch/2
  Constant2/1 -> Switch/3
  Constant1/1 -> Switch/1

== system spike_generator/4-Site Synaptic Release & Adaptive Redocking/Redock Site Original/Redock Component/Initialization Signal1 ==
  note: This should probably be a model reference...
  Constant1 : Constant  Value=0  SampleTime=-1
  Constant2 : Constant  SampleTime=-1
  Data Type Conversion : DataTypeConversion  OutDataTypeStr=boolean
  HDL Counter : hdlsllib/Sources/HDL Counter  CountType=Count limited  CountInit=0  CountStep=1  CountMax=2  CountFromType=Initial value  CountFrom=0  CountResetPort=off  CountLoadPort=off  CountEnbPort=on  CountDirPort=off  CountDataType=Unsigned  CountWordLen=2  CountFracLen=0  CountSampTime=-1
  Switch : Switch  Criteria=u2 > Threshold
  initalize : Outport
  wires:
  Data Type Conversion/1 -> HDL Counter/1
  Switch/1 -> initalize/1, Data Type Conversion/1
  HDL Counter/1 -> Switch/2
  Constant2/1 -> Switch/3
  Constant1/1 -> Switch/1

== system spike_generator/4-Site Synaptic Release & Adaptive Redocking/Redocking Calculation/Current Redock Component/Initialization Signal ==
  note: This should probably be a model reference...
  Constant1 : Constant  Value=0  SampleTime=-1
  Constant2 : Constant  SampleTime=-1
  Data Type Conversion : DataTypeConversion  OutDataTypeStr=boolean
  HDL Counter : hdlsllib/Sources/HDL Counter  CountType=Count limited  CountInit=0  CountStep=1  CountMax=3  CountFromType=Initial value  CountFrom=0  CountResetPort=off  CountLoadPort=off  CountEnbPort=on  CountDirPort=off  CountDataType=Unsigned  CountWordLen=2  CountFracLen=0  CountSampTime=-1
  Switch : Switch  Criteria=u2 > Threshold
  initalize : Outport
  wires:
  Data Type Conversion/1 -> HDL Counter/1
  Switch/1 -> initalize/1, Data Type Conversion/1
  HDL Counter/1 -> Switch/2
  Constant2/1 -> Switch/3
  Constant1/1 -> Switch/1
